simulink subsystem "Vision_Corrections_sub"  (R2023b)
settings: Solver=VariableStepAuto  StartTime=0.0  StopTime=10.0  RelTol=1e-3
undefined symbols (not defined in the file): Vision_Object_Angle_Offset, Vision_Object_X_Offset, Vision_Object_Y_Offset, Vision_Tag_Angle_Offset, Vision_Tag_X_Offset, Vision_Tag_Y_Offset
libraries: simulink x1
settings Model: Creator=ander  LastModifiedBy=ander

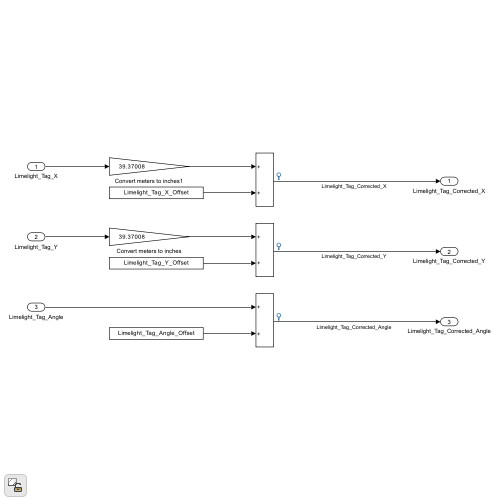
[thumbnail: Simulink's stored preview of the top-level diagram]
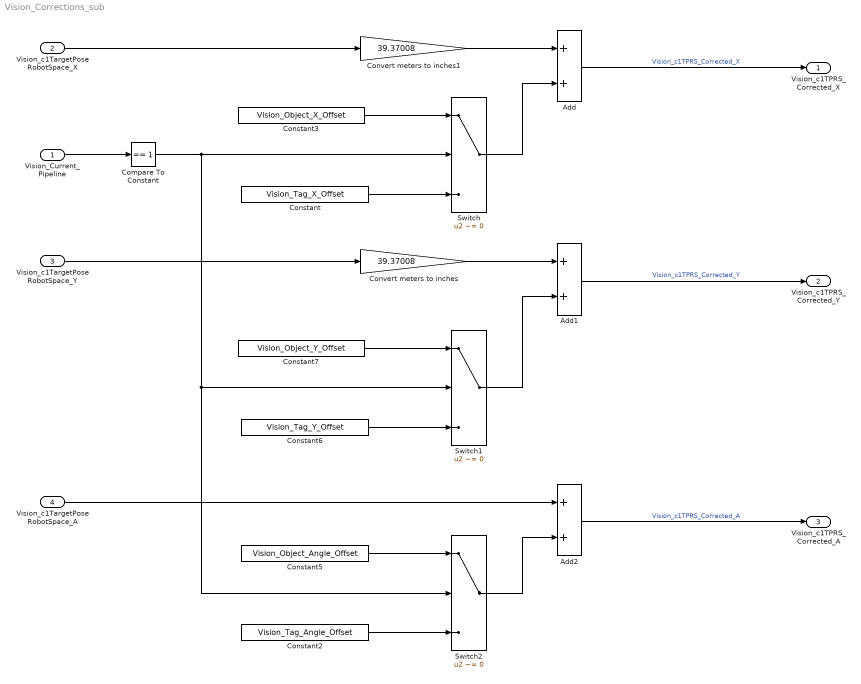
== system Vision_Corrections_sub ==
  Vision_Current_Pipeline : Inport
  Vision_c1TargetPoseRobotSpace_X : Inport  Port=2
  Vision_c1TargetPoseRobotSpace_Y : Inport  Port=3
  Vision_c1TargetPoseRobotSpace_A : Inport  Port=4
  Add : Sum
  Add1 : Sum
  Add2 : Sum
  Compare To Constant : simulink/Logic and Bit Operations/Compare To Constant  relop===  const=1  OutDataTypeStr=boolean
  Constant : Constant  Value=Vision_Tag_X_Offset
  Constant2 : Constant  Value=Vision_Tag_Angle_Offset
  Constant3 : Constant  Value=Vision_Object_X_Offset
  Constant5 : Constant  Value=Vision_Object_Angle_Offset
  Constant6 : Constant  Value=Vision_Tag_Y_Offset
  Constant7 : Constant  Value=Vision_Object_Y_Offset
  Convert meters to inches : Gain  Gain=39.37008
  Convert meters to inches1 : Gain  Gain=39.37008
  Switch : Switch  Criteria=u2 ~= 0  SaturateOnIntegerOverflow=off  InputSameDT=off
  Switch1 : Switch  Criteria=u2 ~= 0  SaturateOnIntegerOverflow=off  InputSameDT=off
  Switch2 : Switch  Criteria=u2 ~= 0  SaturateOnIntegerOverflow=off  InputSameDT=off
  Vision_c1TPRS_Corrected_X : Outport
  Vision_c1TPRS_Corrected_Y : Outport  Port=2
  Vision_c1TPRS_Corrected_A : Outport  Port=3
  wires:
  Convert meters to inches1/1 -> Add/1
  Convert meters to inches/1 -> Add1/1
  Add2/1 -> Vision_c1TPRS_Corrected_A/1  "Vision_c1TPRS_Corrected_A"
  Add1/1 -> Vision_c1TPRS_Corrected_Y/1  "Vision_c1TPRS_Corrected_Y"
  Vision_c1TargetPoseRobotSpace_Y/1 -> Convert meters to inches/1
  Vision_c1TargetPoseRobotSpace_A/1 -> Add2/1
  Add/1 -> Vision_c1TPRS_Corrected_X/1  "Vision_c1TPRS_Corrected_X"
  Vision_c1TargetPoseRobotSpace_X/1 -> Convert meters to inches1/1
  Compare To Constant/1 -> Switch/2, Switch2/2, Switch1/2
  Vision_Current_Pipeline/1 -> Compare To Constant/1
  Constant3/1 -> Switch/1
  Constant/1 -> Switch/3
  Switch/1 -> Add/2
  Constant7/1 -> Switch1/1
  Constant6/1 -> Switch1/3
  Switch1/1 -> Add1/2
  Switch2/1 -> Add2/2
  Constant2/1 -> Switch2/3
  Constant5/1 -> Switch2/1
